simulink library "asbhl20vehicle"  (R2016b)
settings: Solver=ode45  StartTime=0.0  StopTime=10.0  RelTol=1e-3
undefined symbols (not defined in the file): alpha_vec_Cn0, b_ref, beta_vec_Cn0, Clbeta, Clda, Clddf, Cldr, Clp, Clr, Cm0, cm_GE, cm_LG, Cmda, Cmde, Cmdfn, Cmdfp, Cmdr, Cmq, Cn0, Cnda, Cnddf, Cndr, Cnp, Cnr, CX0, cx_GE, cx_LG, CXda, CXddf, CXde, CXdfn, CXdfp, CXdr, CYbeta, CYda, CYddf, CYdr, CZ0, cz_GE, cz_LG, CZda, CZde, CZdfn, CZdfp, CZdr, d_ref, Earth, Euler_0, heading0, LongLat0, mass, Tfg, Tplant, Ts, WGS84, x_cg, x_ref
libraries: aerolibtransform2 x6, aerolibconvert2 x4, aerolibasang x3, aerolibobsolete x3, aerolibutil x3, aerolib6dof2 x1, aerolibadyn x1, asbhl20act x1, discretizing x1
(part 1 of 2)
Description:
  | HL-20 vehicle plant model top component module (continuous)
settings Model: ExtModeAutoUpdateStatusClock=off  Creator=The MathWorks, Inc.  LastModifiedBy=The MathWorks, Inc.
settings DataIOCC: LimitDataPoints=on  SaveFormat=Array  SignalLoggingSaveFormat=ModelDataLogs
settings OptimizationCC: BlockReduction=off  BooleanDataType=off  ExpressionDepthLimit=2147483647  LifeSpan=inf
settings DebuggingCC: SaveWithParameterizedLinksMsg=none  UnderspecifiedInitializationDetection=Classic  MergeDetectMultiDrivingBlocksExec=none  SignalResolutionControl=TryResolveAllWithWarning  FcnCallInpInsideContextMsg=warning  StateNameClashWarn=warning  StrictBusMsg=Warning  SFUnexpectedBacktrackingDiag=warning  SFNoUnconditionalDefaultTransitionDiag=warning  SFExecutionAtInitializationDiag=none
settings HardwareCC: ProdBitPerPointer=32  ProdBitPerSizeT=32  ProdBitPerPtrDiffT=32  ProdLargestAtomicFloat=None  ProdIntDivRoundTo=Undefined  ProdEndianess=Unspecified  ProdWordSize=32  ProdHWDeviceType=32-bit Generic  TargetUnknown=on
settings ModelReferenceCC: PropagateSignalLabelsOutOfModel=off
settings GRTTargetCC: TargetLangStandard=C89/C90 (ANSI)  GeneratePreprocessorConditionals=Disable all  CombineOutputUpdateFcns=off  GRTInterface=on
settings ConfigComp: CovMetricSettings=dw  CovHtmlReporting=on  CovSaveCumulativeToWorkspaceVar=on  CovSaveSingleToWorkspaceVar=on  CovExternalEMLEnable=off

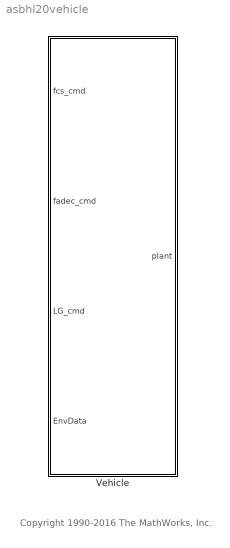
== system asbhl20vehicle ==
  note: Copyright 1990-2016 The MathWorks, Inc.
  Vehicle : Subsystem

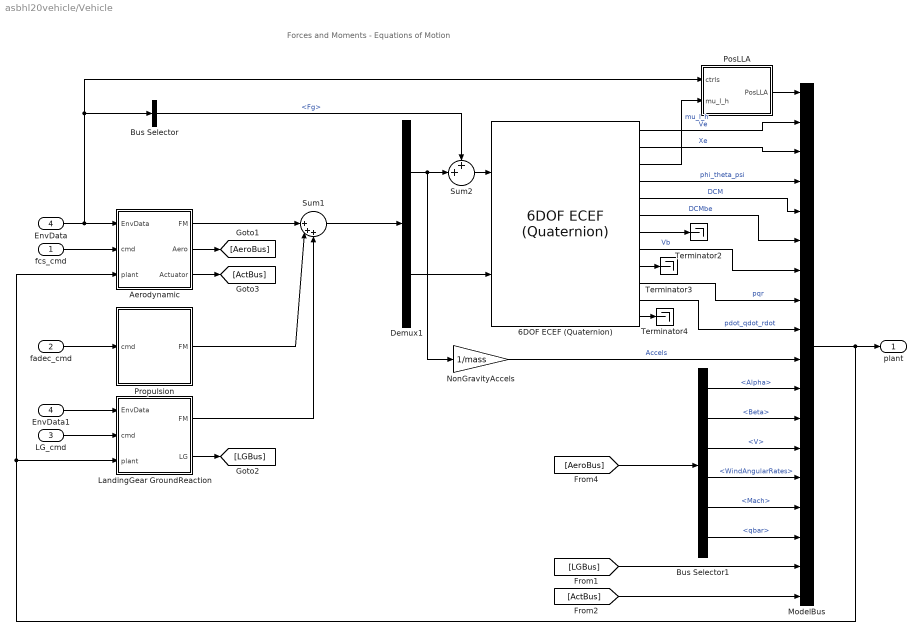
== system asbhl20vehicle/Vehicle ==
  note: Forces and Moments - Equations of Motion
  fcs_cmd : Inport
  fadec_cmd : Inport  Port=2
  LG_cmd : Inport  Port=3
  EnvData : Inport  Port=4
  6DOF ECEF (Quaternion) : aerolib6dof2/6DOF ECEF (Quaternion)  units=Metric (MKS)  mtype=Fixed  xg_0="[LongLat0(2)  LongLat0(1) 2275.5]"  Vm_0=Vmw  eul_0=[Euler_0(1) Euler_0(2) Euler_0(3)+heading0*pi/180]  pm_0=pm_0  mass_0=mass  mass_e=0.5  mass_f=2.0  inertia=Inertia  inertia_e=eye(3)  inertia_f=2*eye(3)  vre_flag=on  ptype=Earth (WGS84)  R=6378137  F=1/298.257223563  w_E=7292115e-11  angle_in=Internal  LG0=0
  Aerodynamic : Subsystem
  Bus Selector : BusSelector  OutputSignals=Fg
  Bus Selector1 : BusSelector  OutputSignals=Alpha,Beta,V,WindAngularRates,Mach,qbar
  Demux1 : Demux  Outputs=[3,3]
  EnvData1 : InportShadow  Port=4
  LandingGear GroundReaction : Subsystem
  ModelBus : BusCreator  Inputs='PosLLA','Ve','Xe','phi_theta_psi','DCM','DCMbe','Vb','pqr','pdot_qdot_rdot','Accels','Alpha','Beta','V','WindAngularRates','Mach','qbar','LGData','Act_positions'
  NonGravityAccels : Gain  Gain=1/mass  SaturateOnIntegerOverflow=on  OutDataTypeStr=Inherit: Same as input  ParamDataTypeStr=Inherit: Same as input
  PosLLA : Subsystem
  Propulsion : Subsystem  SystemSampleTime=Tfg
      settings: RTWSystemCode=Inline
  Sum1 : Sum  Inputs=||+++  SaturateOnIntegerOverflow=on  InputSameDT=on  OutDataTypeStr=Inherit: Same as first input
  Sum2 : Sum  Inputs=++|  SaturateOnIntegerOverflow=on  InputSameDT=on  OutDataTypeStr=Inherit: Same as first input
  Terminator2 : Terminator
  Terminator3 : Terminator
  Terminator4 : Terminator
  plant : Outport
  wires:
  PosLLA/1(PosLLA) -> ModelBus/1
  6DOF ECEF (Quaternion)/11 -> ModelBus/9  "pdot_qdot_rdot"
  6DOF ECEF (Quaternion)/12 -> Terminator4/1
  6DOF ECEF (Quaternion)/9 -> Terminator3/1
  6DOF ECEF (Quaternion)/10 -> ModelBus/8  "pqr"
  6DOF ECEF (Quaternion)/8 -> ModelBus/7  "Vb"
  6DOF ECEF (Quaternion)/7 -> Terminator2/1
  6DOF ECEF (Quaternion)/6 -> ModelBus/6  "DCMbe"
  6DOF ECEF (Quaternion)/5 -> ModelBus/5  "DCM"
  6DOF ECEF (Quaternion)/4 -> ModelBus/4  "phi_theta_psi"
  6DOF ECEF (Quaternion)/2 -> ModelBus/3  "Xe"
  6DOF ECEF (Quaternion)/1 -> ModelBus/2  "Ve"
  6DOF ECEF (Quaternion)/3 -> PosLLA/2(mu_l_h)  "mu_l_h"
  EnvData1/1 -> LandingGear GroundReaction/1(EnvData)
  Demux1/2 -> 6DOF ECEF (Quaternion)/2
  Aerodynamic/1(FM) -> Sum1/1
  LandingGear GroundReaction/1(FM) -> Sum1/3
  Sum1/1 -> Demux1/1
  EnvData/1 -> PosLLA/1(ctrls), Bus Selector/1, Aerodynamic/1(EnvData)
  fcs_cmd/1 -> Aerodynamic/2(cmd)
  fadec_cmd/1 -> Propulsion/1(cmd)
  Demux1/1 -> Sum2/2, NonGravityAccels/1
  Sum2/1 -> 6DOF ECEF (Quaternion)/1
  Bus Selector/1 -> Sum2/1  "<Fg>"
  NonGravityAccels/1 -> ModelBus/10  "Accels"
  Aerodynamic/2(Aero) -> [AeroBus]
  [AeroBus] -> Bus Selector1/1
  Bus Selector1/1 -> ModelBus/11  "<Alpha>"
  Bus Selector1/2 -> ModelBus/12  "<Beta>"
  Bus Selector1/3 -> ModelBus/13  "<V>"
  Bus Selector1/4 -> ModelBus/14  "<WindAngularRates>"
  Bus Selector1/5 -> ModelBus/15  "<Mach>"
  Bus Selector1/6 -> ModelBus/16  "<qbar>"
  LandingGear GroundReaction/2(LG) -> [LGBus]
  [LGBus] -> ModelBus/17
  LG_cmd/1 -> LandingGear GroundReaction/2(cmd)
  ModelBus/1 -> plant/1, Aerodynamic/3(plant), LandingGear GroundReaction/3(plant)
  Aerodynamic/3(Actuator) -> [ActBus]
  [ActBus] -> ModelBus/18
  Propulsion/1(FM) -> Sum1/2

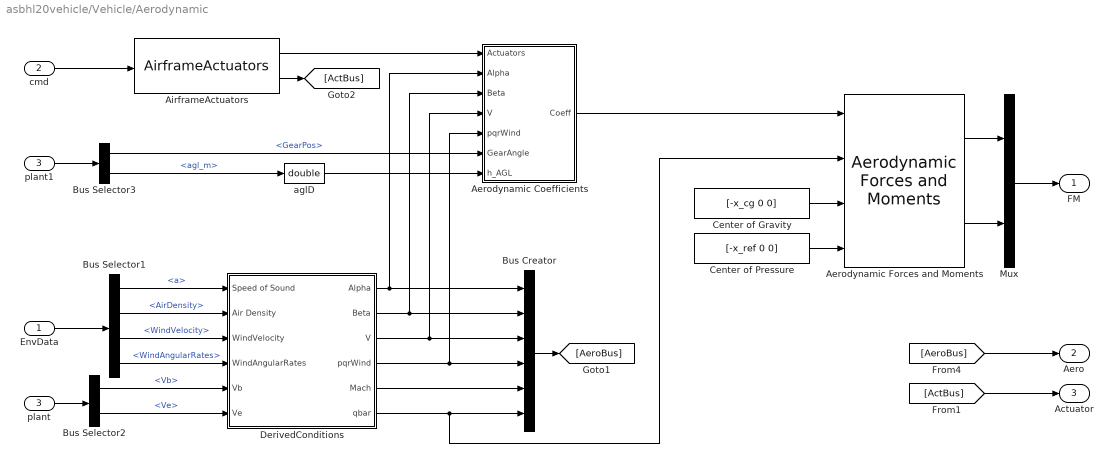
== system asbhl20vehicle/Vehicle/Aerodynamic ==
  EnvData : Inport
  cmd : Inport  Port=2
  plant : Inport  Port=3
  Aerodynamic Coefficients : Subsystem
  Aerodynamic Forces and Moments : aerolibadyn/Aerodynamic Forces and Moments   inputAxes=Body  outputForceAxes=Body  outputMomentAxes=Body  S=S_ref  b=b_ref  cbar=d_ref
  AirframeActuators : asbhl20act/AirframeActuators
  Bus Creator : BusCreator  Inputs='Alpha','Beta','V','WindAngularRates','Mach','qbar'
  Bus Selector1 : BusSelector  OutputSignals=a,AirDensity,WindVelocity,WindAngularRates
  Bus Selector2 : BusSelector  OutputSignals=Vb,Ve
  Bus Selector3 : BusSelector  OutputSignals=LGData.GearPos,PosLLA.agl_m
  Center of Gravity : Constant  Value=[-x_cg 0 0]  SampleTime=0
  Center of Pressure : Constant  Value=[-x_ref 0 0]  SampleTime=0
  DerivedConditions : Subsystem
  Mux : Mux  Inputs=2
  aglD : DataTypeConversion  OutDataTypeStr=double  SaturateOnIntegerOverflow=on
  plant1 : InportShadow  Port=3
  FM : Outport  PortDimensions=6  InitialOutput=0
  Aero : Outport  Port=2  InitialOutput=0
  Actuator : Outport  Port=3  InitialOutput=0
  wires:
  Center of Pressure/1 -> Aerodynamic Forces and Moments/4
  Center of Gravity/1 -> Aerodynamic Forces and Moments/3
  Bus Selector3/1 -> Aerodynamic Coefficients/6(GearAngle)  "<GearPos>"
  Bus Selector3/2 -> aglD/1  "<agl_m>"
  plant1/1 -> Bus Selector3/1
  cmd/1 -> AirframeActuators/1
  Aerodynamic Coefficients/1(Coeff) -> Aerodynamic Forces and Moments/1
  Aerodynamic Forces and Moments/1 -> Mux/1
  Aerodynamic Forces and Moments/2 -> Mux/2
  Mux/1 -> FM/1
  DerivedConditions/1(Alpha) -> Bus Creator/1, Aerodynamic Coefficients/2(Alpha)
  DerivedConditions/2(Beta) -> Bus Creator/2, Aerodynamic Coefficients/3(Beta)
  DerivedConditions/3(V) -> Bus Creator/3, Aerodynamic Coefficients/4(V)
  DerivedConditions/4("pqrWind ") -> Bus Creator/4, Aerodynamic Coefficients/5(pqrWind)
  DerivedConditions/5(Mach) -> Bus Creator/5
  DerivedConditions/6(qbar) -> Aerodynamic Forces and Moments/2, Bus Creator/6
  Bus Creator/1 -> [AeroBus]
  [AeroBus] -> Aero/1
  EnvData/1 -> Bus Selector1/1
  Bus Selector1/1 -> DerivedConditions/1(Speed of Sound)  "<a>"
  Bus Selector1/2 -> DerivedConditions/2(Air Density)  "<AirDensity>"
  plant/1 -> Bus Selector2/1
  Bus Selector1/3 -> DerivedConditions/3(WindVelocity)  "<WindVelocity>"
  Bus Selector1/4 -> DerivedConditions/4(WindAngularRates)  "<WindAngularRates>"
  AirframeActuators/1 -> Aerodynamic Coefficients/1(Actuators)
  Bus Selector2/1 -> DerivedConditions/5(Vb)  "<Vb>"
  Bus Selector2/2 -> DerivedConditions/6(Ve)  "<Ve>"
  aglD/1 -> Aerodynamic Coefficients/7(h_AGL)
  AirframeActuators/2 -> [ActBus]
  [ActBus] -> Actuator/1

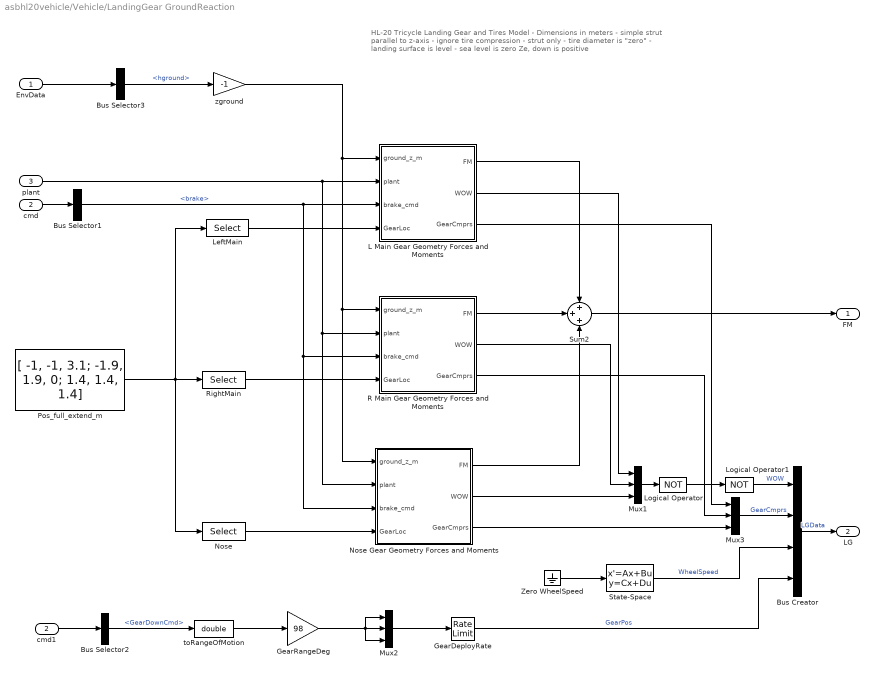
== system asbhl20vehicle/Vehicle/LandingGear GroundReaction ==
  note: HL-20 Tricycle Landing Gear and Tires Model
      |  - Dimensions in meters
      |  - simple strut parallel to z-axis
      |  - ignore tire compression - strut only
      |  - tire diameter is "zero"
      |  - landing surface is level
      |  - sea level is zero Ze, down is positive
  EnvData : Inport  SampleTime=Ts
  cmd : Inport  Port=2
  plant : Inport  Port=3
  Bus Creator : BusCreator  Inputs=4
  Bus Selector1 : BusSelector  OutputSignals=brake
  Bus Selector2 : BusSelector  OutputSignals=GearDownCmd
  Bus Selector3 : BusSelector  OutputSignals=hground
  GearDeployRate : RateLimiter  RisingSlewLimit=50  FallingSlewLimit=-50  SampleTimeMode=inherited
      settings: AttributesFormatString=[%<RisingSlewLimit>, %<FallingSlewLimit>] deg_per_sec
  GearRangeDeg : Gain  Gain=98
  L Main Gear Geometry Forces and Moments : Subsystem  TreatAsAtomicUnit=on
  LeftMain : Selector  NumberOfDimensions=2  InputPortWidth=3  IndexOptions=Select all,Index vector (dialog)  Indices=-1,1  OutputSizes=1
  Logical Operator : Logic  Operator=NOT  IconShape=distinctive  AllPortsSameDT=off  OutDataTypeStr=boolean
  Logical Operator1 : Logic  Operator=NOT  IconShape=distinctive  AllPortsSameDT=off  OutDataTypeStr=boolean
  Mux1 : Mux  Inputs=3
  Mux2 : Mux  Inputs=3
  Mux3 : Mux  Inputs=3
  Nose : Selector  NumberOfDimensions=2  InputPortWidth=3  IndexOptions=Select all,Index vector (dialog)  Indices=-1,3  OutputSizes=1
  Nose Gear Geometry Forces and Moments : Subsystem  TreatAsAtomicUnit=on
  Pos_full_extend_m : Constant  Description=|  Value=[ -1, -1, 3.1; -1.9, 1.9, 0; 1.4, 1.4, 1.4]
      | Rows are X, Y, Z; cols are Left, Right, Nose gear
      | Measured from CG in meters
      settings: AttributesFormatString=%<Description>
  R Main Gear Geometry Forces and Moments : Subsystem  TreatAsAtomicUnit=on
  RightMain : Selector  NumberOfDimensions=2  InputPortWidth=3  IndexOptions=Select all,Index vector (dialog)  Indices=-1,2  OutputSizes=1
  State-Space : StateSpace  A=[]  B=[]  C=[]  D=[1,1,1]'  X0=0
  Sum2 : Sum  Inputs=+++  SaturateOnIntegerOverflow=on  InputSameDT=on  OutDataTypeStr=Inherit: Same as first input
  Zero WheelSpeed : Ground
  cmd1 : InportShadow  Port=2
  toRangeOfMotion : DataTypeConversion  OutDataTypeStr=double  SampleTime=Tplant
  zground : Gain  Gain=-1
  FM : Outport
  LG : Outport  Port=2
  wires:
  Zero WheelSpeed/1 -> State-Space/1
  Logical Operator1/1 -> Bus Creator/1  "WOW"
  Logical Operator/1 -> Logical Operator1/1
  State-Space/1 -> Bus Creator/3  "WheelSpeed"
  Nose Gear Geometry Forces and Moments/3(GearCmprs) -> Mux3/3
  Mux3/1 -> Bus Creator/2  "GearCmprs"
  GearDeployRate/1 -> Bus Creator/4  "GearPos"
  R Main Gear Geometry Forces and Moments/3(GearCmprs) -> Mux3/2
  L Main Gear Geometry Forces and Moments/3(GearCmprs) -> Mux3/1
  Mux2/1 -> GearDeployRate/1
  GearRangeDeg/1 -> Mux2/3, Mux2/2, Mux2/1
  toRangeOfMotion/1 -> GearRangeDeg/1
  Bus Selector2/1 -> toRangeOfMotion/1  "<GearDownCmd>"
  cmd1/1 -> Bus Selector2/1
  Nose/1 -> Nose Gear Geometry Forces and Moments/4(GearLoc)
  Bus Selector1/1 -> Nose Gear Geometry Forces and Moments/3(brake_cmd), R Main Gear Geometry Forces and Moments/3(brake_cmd), L Main Gear Geometry Forces and Moments/3(brake_cmd)  "<brake>"
  RightMain/1 -> R Main Gear Geometry Forces and Moments/4(GearLoc)
  L Main Gear Geometry Forces and Moments/1(FM) -> Sum2/1
  Nose Gear Geometry Forces and Moments/2(WOW) -> Mux1/3
  R Main Gear Geometry Forces and Moments/2(WOW) -> Mux1/2
  L Main Gear Geometry Forces and Moments/2(WOW) -> Mux1/1
  Nose Gear Geometry Forces and Moments/1(FM) -> Sum2/3
  Sum2/1 -> FM/1
  R Main Gear Geometry Forces and Moments/1(FM) -> Sum2/2
  LeftMain/1 -> L Main Gear Geometry Forces and Moments/4(GearLoc)
  Pos_full_extend_m/1 -> LeftMain/1, Nose/1, RightMain/1
  zground/1 -> L Main Gear Geometry Forces and Moments/1(ground_z_m), Nose Gear Geometry Forces and Moments/1(ground_z_m), R Main Gear Geometry Forces and Moments/1(ground_z_m)
  Bus Selector3/1 -> zground/1  "<hground>"
  Mux1/1 -> Logical Operator/1
  cmd/1 -> Bus Selector1/1
  EnvData/1 -> Bus Selector3/1
  Bus Creator/1 -> LG/1  "LGData"
  plant/1 -> Nose Gear Geometry Forces and Moments/2(plant), R Main Gear Geometry Forces and Moments/2(plant), L Main Gear Geometry Forces and Moments/2(plant)

== system asbhl20vehicle/Vehicle/PosLLA ==
  ctrls : Inport
  mu_l_h : Inport  Port=2
  Bus Selector : BusSelector  OutputSignals=hground
  Demux1 : Demux  Outputs=2
  Demux2 : Demux  Outputs=[2 1]
  FilteredROC : discretizing/Discretized Transfer Fcn  Numerator=[1 0]  Denominator=[1 1]  AbsTol=auto  SampleTime=1.0  method=tustin  Wc=1
  ModelBus : BusCreator  Inputs='long_rad','lat_rad','agl_m','alt_m','roc_fps'
  Sel : Selector  InputPortWidth=2  IndexOptions=Index vector (dialog)  Indices=[2 1]  OutputSizes=1
  Sum1 : Sum  Inputs=-+|
  altm : DataTypeConversion  OutDataTypeStr=single  SaturateOnIntegerOverflow=on
  m2ft : aerolibconvert2/Length Conversion  IU=m  OU=ft
  pos_rad : aerolibconvert2/Angle Conversion  IU=deg  OU=rad
  rocF : DataTypeConversion  OutDataTypeStr=single  SaturateOnIntegerOverflow=on
  PosLLA : Outport
  wires:
  altm/1 -> Sum1/2
  Sum1/1 -> ModelBus/3  "agl_m"
  Bus Selector/1 -> Sum1/1  "<hground>"
  ctrls/1 -> Bus Selector/1
  Sel/1 -> pos_rad/1
  Demux2/1 -> Sel/1
  pos_rad/1 -> Demux1/1
  Demux1/1 -> ModelBus/1  "long_rad"
  Demux1/2 -> ModelBus/2  "lat_rad"
  Demux2/2 -> altm/1, m2ft/1, ModelBus/4  "alt_m"
  rocF/1 -> ModelBus/5  "roc_fps"
  mu_l_h/1 -> Demux2/1
  ModelBus/1 -> PosLLA/1  "PosLLA"
  m2ft/1 -> FilteredROC/1
  FilteredROC/1 -> rocF/1

== system asbhl20vehicle/Vehicle/Propulsion ==
  note: HL-20 Propulsion Model
      |   - Thrusters not modeled
  cmd : Inport  SampleTime=Ts
  Mux : Mux  Inputs=3
  SigCat : SignalConversion  ConversionOutput=Contiguous copy  OverrideOpt=off
  ThrustX : Lookup_n-D  NumberOfTableDimensions=1  BreakpointsForDimension1=(1/6)*(3+([-3:3]))  IndexSearchMethod=Linear search  BeginIndexSearchUsingPreviousIndexResult=on  Table=10000*(1+tanh([-3:3]))  ExtrapMethod=Clip  InputSameDT=on
  Thrust_LMN : Constant  Value=[0, 0, 0]  SampleTime=Ts
  Thrust_YZ : Constant  Value=[0, 0]  SampleTime=Ts
  FM : Outport  PortDimensions=6
  wires:
  ThrustX/1 -> Mux/1
  Thrust_YZ/1 -> Mux/2
  Mux/1 -> SigCat/1
  SigCat/1 -> FM/1
  cmd/1 -> ThrustX/1
  Thrust_LMN/1 -> Mux/3

== system asbhl20vehicle/Vehicle/Aerodynamic/Aerodynamic Coefficients ==
  Actuators : Inport
  Alpha : Inport  Port=2
  Beta : Inport  Port=3
  V : Inport  Port=4
  pqrWind : Inport  Port=5
  GearAngle : Inport  Port=6
  h_AGL : Inport  Port=7
  Actuator Increments : Subsystem
  Body Rate Damping : Subsystem
  Datum Coefficients : Subsystem
  Ground Effects : Subsystem
  Landing Gear Effects : Subsystem
  Sum1 : Sum  Inputs=+++  SaturateOnIntegerOverflow=on  InputSameDT=on  OutDataTypeStr=Inherit: Same as first input
  Sum2 : Sum  Inputs=+++  SaturateOnIntegerOverflow=on  InputSameDT=on  OutDataTypeStr=Inherit: Same as first input
  alpha_rad : aerolibconvert2/Angle Conversion  IU=rad  OU=deg
  beta_rad : aerolibconvert2/Angle Conversion  IU=rad  OU=deg
  on_off1 : Gain
  on_off2 : Gain
  Coeff : Outport  InitialOutput=0
  wires:
  on_off1/1 -> Sum2/3
  on_off2/1 -> Sum2/2
  Ground Effects/1(Coeff) -> on_off1/1
  Landing Gear Effects/1(Coeff) -> on_off2/1
  Sum1/1 -> Sum2/1
  Sum2/1 -> Coeff/1
  GearAngle/1 -> Landing Gear Effects/3(Landing Gear Angle)
  h_AGL/1 -> Ground Effects/3(h_AGL)
  Body Rate Damping/1(cl) -> Sum1/3
  Actuator Increments/1(cl) -> Sum1/1
  V/1 -> Body Rate Damping/1(V)
  Beta/1 -> beta_rad/1
  beta_rad/1 -> Ground Effects/2(Beta), Landing Gear Effects/2(Beta), Datum Coefficients/2(Beta), Actuator Increments/2(Beta)
  Datum Coefficients/1(cl) -> Sum1/2
  Actuators/1 -> Actuator Increments/3("Actuator Deflections ")
  Alpha/1 -> alpha_rad/1
  pqrWind/1 -> Body Rate Damping/2(p,q,r)
  alpha_rad/1 -> Ground Effects/1(Alpha), Landing Gear Effects/1(Alpha), Body Rate Damping/3(Alpha), Datum Coefficients/1(Alpha), Actuator Increments/1(Alpha)

== system asbhl20vehicle/Vehicle/Aerodynamic/DerivedConditions ==
  note: TODO: clean up interface
  Speed of Sound : Inport
  Air Density : Inport  Port=2
  WindVelocity : Inport  Port=3  PortDimensions=3
  WindAngularRates : Inport  Port=4  PortDimensions=3
  Vb : Inport  Port=5  PortDimensions=3
  Ve : Inport  Port=6  PortDimensions=3
  Dynamic Pressure : aerolibasang/Dynamic Pressure
  "Incidence, Sideslip, & Airspeed" : aerolibasang/Incidence, Sideslip, & Airspeed
  Mach Number : aerolibasang/Mach Number
  Sum2 : Sum  Inputs=|+-  SaturateOnIntegerOverflow=on  InputSameDT=on  OutDataTypeStr=Inherit: Same as first input
  Terminator : Terminator
  Alpha : Outport
  Beta : Outport  Port=2
  V : Outport  Port=3
  "pqrWind " : Outport  Port=4
  Mach : Outport  Port=5
  qbar : Outport  Port=6  InitialOutput=0
  wires:
  "Incidence, Sideslip, & Airspeed"/1 -> Alpha/1  "Alpha"
  "Incidence, Sideslip, & Airspeed"/2 -> Beta/1  "Beta"
  Speed of Sound/1 -> Mach Number/2
  "Incidence, Sideslip, & Airspeed"/3 -> V/1  "V"
  Mach Number/1 -> Mach/1  "Mach"
  Air Density/1 -> Dynamic Pressure/2
  Dynamic Pressure/1 -> qbar/1  "qbar"
  WindAngularRates/1 -> "pqrWind "/1
  Vb/1 -> Sum2/1
  Sum2/1 -> Dynamic Pressure/1, Mach Number/1, "Incidence, Sideslip, & Airspeed"/1
  WindVelocity/1 -> Sum2/2
  Ve/1 -> Terminator/1

== system asbhl20vehicle/Vehicle/LandingGear GroundReaction/L Main Gear Geometry Forces and Moments ==
  note: Gear compression is assumed to occur
      | algebraically in proportion to the amount
      | of fully extended gear that would be
      | "below ground".
  note: HL-20 Tricycle Landing Gear and Tires Model
      |  - Dimensions in meters
      |  - simple strut parallel to z-axis
      |  - ignore tire compression - strut only
      |  - landing surface is level
      |  - sea level is zero Ze, down is positive
  ground_z_m : Inport
  plant : Inport  Port=2
  brake_cmd : Inport  Port=3
  GearLoc : Inport  Port=4
  Bus Selector3 : BusSelector  OutputSignals=PosLLA.alt_m,phi_theta_psi
  GearLoc1 : InportShadow  Port=4
  GenerateGroundFM : Subsystem  TreatAsAtomicUnit=on
  Rotate pos to body axes : Product  Multiplication=Matrix(*)  SaturateOnIntegerOverflow=on  InputSameDT=on  OutDataTypeStr=Inherit: Same as first input
  Subsystem : Subsystem
  Sum3 : Sum  Inputs=-+
  Zg : Selector  InputPortWidth=3  IndexOptions=Index vector (dialog)  Indices=3  OutputSizes=1
  detect_WOW : RelationalOperator  OutDataTypeStr=boolean  RndMeth=Nearest
  FM : Outport  PortDimensions=6
  WOW : Outport  Port=2
  GearCmprs : Outport  Port=3
  wires:
  Bus Selector3/2 -> Subsystem/1(Euler)  "<phi_theta_psi>"
  Zg/1 -> Sum3/2
  GenerateGroundFM/2(GearCmprs) -> GearCmprs/1
  Bus Selector3/1 -> [Xe]  "<alt_m>"
  [ZcL] -> GenerateGroundFM/2(ZcL)
  GenerateGroundFM/1(FM) -> FM/1
  brake_cmd/1 -> GenerateGroundFM/4(BrakeCmd)
  GearLoc1/1 -> Rotate pos to body axes/2
  [DCM] -> Rotate pos to body axes/1
  plant/1 -> Bus Selector3/1, GenerateGroundFM/3(plant)
  GearLoc/1 -> GenerateGroundFM/5(GearLoc)
  ground_z_m/1 -> detect_WOW/2, GenerateGroundFM/1(ground_z)
  detect_WOW/1 -> WOW/1, GenerateGroundFM/Enable
  Rotate pos to body axes/1 -> Zg/1
  Sum3/1 -> detect_WOW/1
  [Xe] -> [ZcL], Sum3/1
  Subsystem/1(DCM) -> [DCM]

== system asbhl20vehicle/Vehicle/LandingGear GroundReaction/Nose Gear Geometry Forces and Moments ==
  note: Gear compression is assumed to occur
      | algebraically in proportion to the amount
      | of fully extended gear that would be
      | "below ground".
  note: HL-20 Tricycle Landing Gear and Tires Model
      |  - Dimensions in meters
      |  - simple strut parallel to z-axis
      |  - ignore tire compression - strut only
      |  - landing surface is level
      |  - sea level is zero Ze, down is positive
  ground_z_m : Inport
  plant : Inport  Port=2
  brake_cmd : Inport  Port=3
  GearLoc : Inport  Port=4
  Bus Selector3 : BusSelector  OutputSignals=PosLLA.alt_m,phi_theta_psi
  GearLoc1 : InportShadow  Port=4
  GenerateGroundFM : Subsystem  TreatAsAtomicUnit=on
  Rotate pos to body axes : Product  Multiplication=Matrix(*)  SaturateOnIntegerOverflow=on  InputSameDT=on  OutDataTypeStr=Inherit: Same as first input
  Subsystem : Subsystem
  Sum3 : Sum  Inputs=-+
  Zg : Selector  InputPortWidth=3  IndexOptions=Index vector (dialog)  Indices=3  OutputSizes=1
  detect_WOW : RelationalOperator  OutDataTypeStr=boolean  RndMeth=Nearest
  FM : Outport  PortDimensions=6
  WOW : Outport  Port=2
  GearCmprs : Outport  Port=3
  wires:
  Zg/1 -> Sum3/2
  GenerateGroundFM/2(GearCmprs) -> GearCmprs/1
  Bus Selector3/1 -> [Xe]  "<alt_m>"
  [ZcL] -> GenerateGroundFM/2(ZcL)
  GenerateGroundFM/1(FM) -> FM/1
  brake_cmd/1 -> GenerateGroundFM/4(BrakeCmd)
  GearLoc1/1 -> Rotate pos to body axes/2
  [DCM] -> Rotate pos to body axes/1
  plant/1 -> Bus Selector3/1, GenerateGroundFM/3(plant)
  GearLoc/1 -> GenerateGroundFM/5(GearLoc)
  ground_z_m/1 -> GenerateGroundFM/1(ground_z), detect_WOW/2
  detect_WOW/1 -> GenerateGroundFM/Enable, WOW/1
  Rotate pos to body axes/1 -> Zg/1
  Sum3/1 -> detect_WOW/1
  [Xe] -> [ZcL], Sum3/1
  Bus Selector3/2 -> Subsystem/1(Euler)  "<phi_theta_psi>"
  Subsystem/1(DCM) -> [DCM]

== system asbhl20vehicle/Vehicle/LandingGear GroundReaction/R Main Gear Geometry Forces and Moments ==
  note: HL-20 Tricycle Landing Gear and Tires Model
      |  - Dimensions in meters
      |  - simple strut parallel to z-axis
      |  - ignore tire compression - strut only
      |  - landing surface is level
      |  - sea level is zero Ze, down is positive
  note: Gear compression is assumed to occur
      | algebraically in proportion to the amount
      | of fully extended gear that would be
      | "below ground".
  ground_z_m : Inport
  plant : Inport  Port=2
  brake_cmd : Inport  Port=3
  GearLoc : Inport  Port=4
  Bus Selector3 : BusSelector  OutputSignals=PosLLA.alt_m,phi_theta_psi
  GearLoc1 : InportShadow  Port=4
  GenerateGroundFM : Subsystem  TreatAsAtomicUnit=on
  Rotate pos to body axes : Product  Multiplication=Matrix(*)  SaturateOnIntegerOverflow=on  InputSameDT=on  OutDataTypeStr=Inherit: Same as first input
  Subsystem1 : Subsystem
  Sum3 : Sum  Inputs=-+
  Zg : Selector  InputPortWidth=3  IndexOptions=Index vector (dialog)  Indices=3  OutputSizes=1
  detect_WOW : RelationalOperator  OutDataTypeStr=boolean  RndMeth=Nearest
  FM : Outport  PortDimensions=6
  WOW : Outport  Port=2
  GearCmprs : Outport  Port=3
  wires:
  Subsystem1/1(DCM) -> [DCM]
  Zg/1 -> Sum3/2
  [Xe] -> [ZcL], Sum3/1
  Sum3/1 -> detect_WOW/1
  Rotate pos to body axes/1 -> Zg/1
  detect_WOW/1 -> GenerateGroundFM/Enable, WOW/1
  ground_z_m/1 -> detect_WOW/2, GenerateGroundFM/1(ground_z)
  GearLoc/1 -> GenerateGroundFM/5(GearLoc)
  plant/1 -> GenerateGroundFM/3(plant), Bus Selector3/1
  [DCM] -> Rotate pos to body axes/1
  GearLoc1/1 -> Rotate pos to body axes/2
  brake_cmd/1 -> GenerateGroundFM/4(BrakeCmd)
  GenerateGroundFM/1(FM) -> FM/1
  [ZcL] -> GenerateGroundFM/2(ZcL)
  Bus Selector3/1 -> [Xe]  "<alt_m>"
  GenerateGroundFM/2(GearCmprs) -> GearCmprs/1
  Bus Selector3/2 -> Subsystem1/1(Euler)  "<phi_theta_psi>"

== system asbhl20vehicle/Vehicle/Aerodynamic/Aerodynamic Coefficients/Actuator Increments ==
  Alpha : Inport
  Beta : Inport  Port=2
  "Actuator Deflections " : Inport  Port=3
  (0 to inf) Constants Held fixed for alpha<0 : Saturate  UpperLimit=inf  LowerLimit=0
  Aileron : Subsystem
  AlphaLookup : PreLookup  BreakpointsData=alpha_vec_0  BeginIndexSearchUsingPreviousIndexResult=on  ExtrapMethod=Linear
  AlphaLookup0 : PreLookup  BreakpointsData=alpha_vec_0  BeginIndexSearchUsingPreviousIndexResult=on  ExtrapMethod=Linear
  Bus Creator : BusCreator  Inputs=2
  Bus Creator1 : BusCreator  Inputs=2
  Elevator : Subsystem
  Flap(diff) : Subsystem
  Flap(neg) : Subsystem
  Flap(pos) : Subsystem
  Rudder : Subsystem
  Sum : Sum  Inputs=++++++  SaturateOnIntegerOverflow=on  InputSameDT=on  OutDataTypeStr=Inherit: Same as first input
  Terminator1 : Terminator
  cl : Outport  InitialOutput=0
  wires:
  Bus Creator/1 -> Aileron/1(Alpha), Rudder/1(Alpha)
  (0 to inf) Constants Held fixed for alpha<0/1 -> AlphaLookup0/1
  "Actuator Deflections "/1 -> Aileron/2(Actuators), Elevator/2(Actuators), Rudder/2(Actuators), Flap(pos)/2(Actuators), Flap(neg)/2(Actuators), Flap(diff)/2(Actuators)
  Alpha/1 -> (0 to inf) Constants Held fixed for alpha<0/1, AlphaLookup/1
  Beta/1 -> Terminator1/1
  Aileron/1(delCoeff) -> Sum/1
  Elevator/1(delCoeff) -> Sum/2
  Rudder/1(delCoeff) -> Sum/3
  Flap(pos)/1(delCoeff) -> Sum/4
  Flap(neg)/1(delCoeff) -> Sum/5
  Flap(diff)/1(delCoeff) -> Sum/6
  Sum/1 -> cl/1
  Bus Creator1/1 -> Flap(diff)/1(Alpha), Flap(neg)/1(Alpha), Flap(pos)/1(Alpha), Elevator/1(Alpha)
  AlphaLookup0/1 -> Bus Creator/1  "k"
  AlphaLookup0/2 -> Bus Creator/2  "f"
  AlphaLookup/1 -> Bus Creator1/1  "k"
  AlphaLookup/2 -> Bus Creator1/2  "f"

== system asbhl20vehicle/Vehicle/Aerodynamic/Aerodynamic Coefficients/Body Rate Damping ==
  V : Inport
  p,q,r : Inport  Port=2
  Alpha : Inport  Port=3
  AlphaLookup : PreLookup  BreakpointsData=alpha_vec_damping  BeginIndexSearchUsingPreviousIndexResult=on  ExtrapMethod=Linear
  Bus Creator : BusCreator  Inputs=2
  Demux : Demux  Outputs=3
  Product : Product  SaturateOnIntegerOverflow=on  InputSameDT=on  OutDataTypeStr=Inherit: Same as first input
  Product1 : Product  SaturateOnIntegerOverflow=on  InputSameDT=on  OutDataTypeStr=Inherit: Same as first input
  Product2 : Product  SaturateOnIntegerOverflow=on  InputSameDT=on  OutDataTypeStr=Inherit: Same as first input
  Product3 : Product  Inputs=*/  SaturateOnIntegerOverflow=on  InputSameDT=on  OutDataTypeStr=Inherit: Same as first input
  Reference Length : Gain  Gain=d_ref/2  SaturateOnIntegerOverflow=on  OutDataTypeStr=Inherit: Same as input  ParamDataTypeStr=Inherit: Same as input
  Reference Span : Gain  Gain=b_ref/2  SaturateOnIntegerOverflow=on  OutDataTypeStr=Inherit: Same as input  ParamDataTypeStr=Inherit: Same as input
  "Reference Span " : Gain  Gain=b_ref/2  SaturateOnIntegerOverflow=on  OutDataTypeStr=Inherit: Same as input  ParamDataTypeStr=Inherit: Same as input
  Sum1 : Sum  Inputs=+++  SaturateOnIntegerOverflow=on  InputSameDT=on  OutDataTypeStr=Inherit: Same as first input
  p : Subsystem
  q : Subsystem
  r : Subsystem
  cl : Outport  InitialOutput=0
  wires:
  Alpha/1 -> AlphaLookup/1
  p/1(delCoeff) -> Product/1
  q/1(delCoeff) -> Product1/1
  p,q,r/1 -> Demux/1
  Demux/1 -> Product/2  "p"
  Demux/2 -> Product1/2  "q"
  Demux/3 -> Product2/2  "r"
  Sum1/1 -> Product3/1
  V/1 -> Product3/2
  Product3/1 -> cl/1
  Product1/1 -> Reference Length/1
  Product2/1 -> "Reference Span "/1
  Product/1 -> Reference Span/1
  r/1(delCoeff) -> Product2/1
  Bus Creator/1 -> r/1(Alpha), q/1(Alpha), p/1(Alpha)
  Reference Length/1 -> Sum1/2
  Reference Span/1 -> Sum1/1
  "Reference Span "/1 -> Sum1/3
  AlphaLookup/1 -> Bus Creator/1  "k"
  AlphaLookup/2 -> Bus Creator/2  "f"

== system asbhl20vehicle/Vehicle/Aerodynamic/Aerodynamic Coefficients/Datum Coefficients ==
  Alpha : Inport
  Beta : Inport  Port=2
  " Cn" : Lookup_n-D  BreakpointsForDimension1=alpha_vec_Cn0  BreakpointsForDimension2=beta_vec_Cn0  Table=Cn0  InternalRulePriority=Speed  RndMeth=Simplest  InputSameDT=on
  " Beta" : InportShadow  Port=2
  " Beta " : InportShadow  Port=2
  Abs : Abs  SaturateOnIntegerOverflow=on
  "Alpha " : InportShadow
  AlphaLookup : PreLookup  BreakpointsData=alpha_vec_0  BeginIndexSearchUsingPreviousIndexResult=on  ExtrapMethod=Linear
  "Beta " : InportShadow  Port=2
  BetaLookup : PreLookup  BreakpointsData=beta_vec_0  BeginIndexSearchUsingPreviousIndexResult=on  ExtrapMethod=Linear
  Cl : Gain  Gain=Clbeta  SaturateOnIntegerOverflow=on  OutDataTypeStr=Inherit: Same as input  ParamDataTypeStr=Inherit: Same as input
  Cm : Interpolation_n-D  Table=Cm0'  RemoveProtectionIndex=on  SaturateOnIntegerOverflow=on
  Cx : Interpolation_n-D  Table=CX0'  RemoveProtectionIndex=on  SaturateOnIntegerOverflow=on
  Cy : Gain  Gain=CYbeta  SaturateOnIntegerOverflow=on  OutDataTypeStr=Inherit: Same as input  ParamDataTypeStr=Inherit: Same as input
  Cz : Interpolation_n-D  Table=CZ0'  RemoveProtectionIndex=on  SaturateOnIntegerOverflow=on
  Mux1 : Mux  Inputs=6
  Product : Product  SaturateOnIntegerOverflow=on  InputSameDT=on  OutDataTypeStr=Inherit: Same as first input
  Sign : Signum
  cl : Outport  InitialOutput=0
  wires:
  Sign/1 -> Product/2
  " Cn"/1 -> Product/1
  Product/1 -> Mux1/6
  Abs/1 -> " Cn"/2
  Mux1/1 -> cl/1
  Cx/1 -> Mux1/1
  Cz/1 -> Mux1/3
  Cm/1 -> Mux1/5
  Cy/1 -> Mux1/2
  Cl/1 -> Mux1/4
  Alpha/1 -> AlphaLookup/1
  Beta/1 -> BetaLookup/1
  AlphaLookup/1 -> Cz/1, Cm/1, Cx/1
  BetaLookup/1 -> Cz/3, Cx/3, Cm/3
  AlphaLookup/2 -> Cx/2, Cm/2, Cz/2
  "Beta "/1 -> Cy/1
  "Alpha "/1 -> " Cn"/1
  " Beta"/1 -> Abs/1, Sign/1
  " Beta "/1 -> Cl/1
  BetaLookup/2 -> Cz/4, Cx/4, Cm/4

== system asbhl20vehicle/Vehicle/Aerodynamic/Aerodynamic Coefficients/Ground Effects ==
  Alpha : Inport
  Beta : Inport  Port=2
  h_AGL : Inport  Port=3
  AlphaLookup : PreLookup  BreakpointsData=GE_alpha_bp  BeginIndexSearchUsingPreviousIndexResult=on
  AltitudeLookup : PreLookup  BreakpointsData=GE_alt_bp  BeginIndexSearchUsingPreviousIndexResult=on
  Cm : Interpolation_n-D  Table=cm_GE  RemoveProtectionIndex=on  SaturateOnIntegerOverflow=on
  Constant1 : Constant  Value=0
  Constant2 : Constant  Value=0
  Constant3 : Constant  Value=0
  Cx : Interpolation_n-D  Table=cx_GE  RemoveProtectionIndex=on  SaturateOnIntegerOverflow=on
  Cz : Interpolation_n-D  Table=cz_GE  RemoveProtectionIndex=on  SaturateOnIntegerOverflow=on
  Gain : Gain  Gain=1/b_ref  SaturateOnIntegerOverflow=on  OutDataTypeStr=Inherit: Same as input  ParamDataTypeStr=Inherit: Same as input
  Mux1 : Mux  Inputs=6
  Terminator1 : Terminator
  Coeff : Outport
  wires:
  AltitudeLookup/2 -> Cm/4, Cz/4, Cx/4
  AlphaLookup/2 -> Cm/2, Cz/2, Cx/2
  Constant3/1 -> Mux1/6
  Cm/1 -> Mux1/5
  Constant2/1 -> Mux1/4
  Cz/1 -> Mux1/3
  Constant1/1 -> Mux1/2
  Cx/1 -> Mux1/1
  Mux1/1 -> Coeff/1
  h_AGL/1 -> Gain/1
  AlphaLookup/1 -> Cx/1, Cm/1, Cz/1
  Beta/1 -> Terminator1/1
  Alpha/1 -> AlphaLookup/1
  AltitudeLookup/1 -> Cm/3, Cz/3, Cx/3
  Gain/1 -> AltitudeLookup/1

== system asbhl20vehicle/Vehicle/Aerodynamic/Aerodynamic Coefficients/Landing Gear Effects ==
  Alpha : Inport
  Beta : Inport  Port=2
  Landing Gear Angle : Inport  Port=3
  AlphaLookup : PreLookup  BreakpointsData=LG_alpha_bp  BeginIndexSearchUsingPreviousIndexResult=on  ExtrapMethod=Linear
  Cm : Interpolation_n-D  Table=cm_LG  RemoveProtectionIndex=on  SaturateOnIntegerOverflow=on
  Constant1 : Constant  Value=0
  Constant2 : Constant  Value=0
  Constant3 : Constant  Value=0
  Cx : Interpolation_n-D  Table=cx_LG  RemoveProtectionIndex=on  SaturateOnIntegerOverflow=on
  Cz : Interpolation_n-D  Table=cz_LG  RemoveProtectionIndex=on  SaturateOnIntegerOverflow=on
  LGLookup : PreLookup  BreakpointsData=LG_bp  BeginIndexSearchUsingPreviousIndexResult=on  ExtrapMethod=Linear
  Mux1 : Mux  Inputs=6
  Sum of Elements : Sum  Inputs=+
  Terminator1 : Terminator
  avg : Gain  Gain=1/3
  Coeff : Outport
  wires:
  LGLookup/2 -> Cm/4, Cz/4, Cx/4
  AlphaLookup/2 -> Cm/2, Cx/2, Cz/2
  LGLookup/1 -> Cm/3, Cz/3, Cx/3
  Constant3/1 -> Mux1/6
  Cm/1 -> Mux1/5
  Constant2/1 -> Mux1/4
  Cz/1 -> Mux1/3
  Constant1/1 -> Mux1/2
  Cx/1 -> Mux1/1
  Mux1/1 -> Coeff/1
  Landing Gear Angle/1 -> Sum of Elements/1
  AlphaLookup/1 -> Cx/1, Cm/1, Cz/1
  Beta/1 -> Terminator1/1
  Alpha/1 -> AlphaLookup/1
  Sum of Elements/1 -> avg/1
  avg/1 -> LGLookup/1

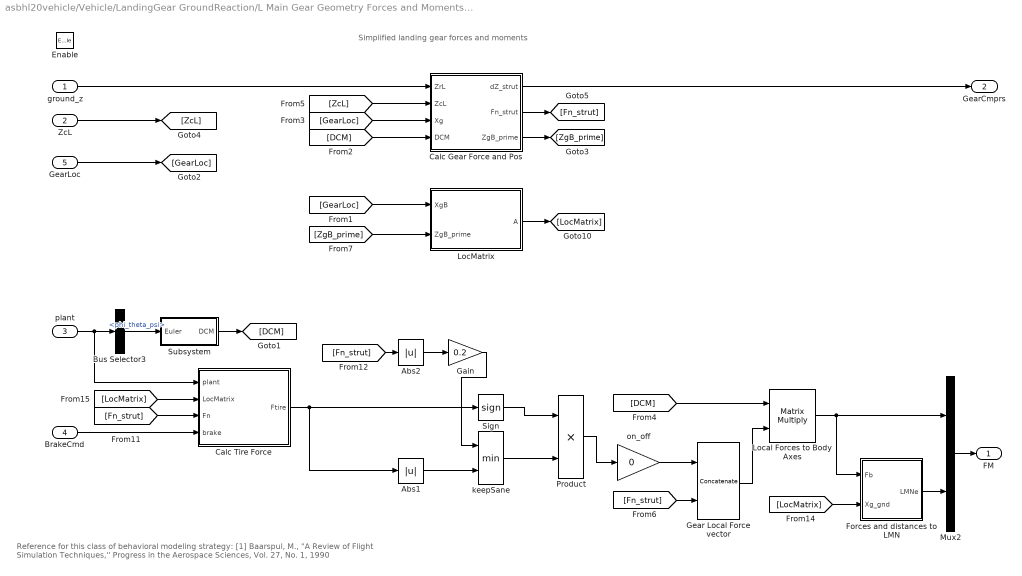
== system asbhl20vehicle/Vehicle/LandingGear GroundReaction/L Main Gear Geometry Forces and Moments/GenerateGroundFM ==
  note: Simplified landing gear forces and moments
  note: Reference for this class of behavioral modeling strategy:
      |
      | [1] Baarspul, M., "A Review of Flight Simulation Techniques,''
      | Progress in the Aerospace Sciences, Vol. 27, No. 1, 1990
  ground_z : Inport
  ZcL : Inport  Port=2
  plant : Inport  Port=3
  BrakeCmd : Inport  Port=4
  GearLoc : Inport  Port=5
  Enable : EnablePort  StatesWhenEnabling=reset
  Abs1 : Abs
  Abs2 : Abs
  Bus Selector3 : BusSelector  OutputSignals=phi_theta_psi
  Calc Gear Force and Pos : Subsystem
  Calc Tire Force : Subsystem
  Forces and distances to LMN : Subsystem
  Gain : Gain  Gain=0.2
  Gear Local Force vector : Concatenate  Mode=Multidimensional array
  LocMatrix : Subsystem
  Local Forces to Body Axes : Product  Multiplication=Matrix(*)  SaturateOnIntegerOverflow=on  InputSameDT=on  OutDataTypeStr=Inherit: Same as first input
  Mux2 : Mux  Inputs=2
  Product : Product  RndMeth=Zero
  Sign : Signum
  Subsystem : Subsystem
  keepSane : MinMax  Inputs=2
  on_off : Gain  Gain=0
  FM : Outport  PortDimensions=6  OutputWhenDisabled=reset  InitialOutput=[0,0,0,0,0,0]
  GearCmprs : Outport  Port=2  OutputWhenDisabled=reset  InitialOutput=0
  wires:
  ZcL/1 -> [ZcL]
  GearLoc/1 -> [GearLoc]
  Mux2/1 -> FM/1
  BrakeCmd/1 -> Calc Tire Force/4(brake)
  plant/1 -> Bus Selector3/1, Calc Tire Force/1(plant)
  ground_z/1 -> Calc Gear Force and Pos/1(ZrL)
  Calc Gear Force and Pos/1(dZ_strut) -> GearCmprs/1
  Sign/1 -> Product/1
  Product/1 -> on_off/1
  keepSane/1 -> Product/2
  Abs1/1 -> keepSane/2
  Gain/1 -> keepSane/1
  Abs2/1 -> Gain/1
  [Fn_strut] -> Abs2/1
  on_off/1 -> Gear Local Force vector/1
  Calc Tire Force/1(Ftire) -> Sign/1, Abs1/1
  [Fn_strut] -> Calc Tire Force/3(Fn)
  [LocMatrix] -> Calc Tire Force/2(LocMatrix)
  [LocMatrix] -> Forces and distances to LMN/2(Xg_gnd)
  LocMatrix/1(A) -> [LocMatrix]
  [ZgB_prime] -> LocMatrix/2(ZgB_prime)
  [GearLoc] -> LocMatrix/1(XgB)
  Forces and distances to LMN/1(LMNe) -> Mux2/2
  Gear Local Force vector/1 -> Local Forces to Body Axes/2
  [Fn_strut] -> Gear Local Force vector/2
  Local Forces to Body Axes/1 -> Mux2/1, Forces and distances to LMN/1(Fb)
  [DCM] -> Local Forces to Body Axes/1
  [DCM] -> Calc Gear Force and Pos/4(DCM)
  [GearLoc] -> Calc Gear Force and Pos/3(Xg)
  Calc Gear Force and Pos/2(Fn_strut) -> [Fn_strut]
  [ZcL] -> Calc Gear Force and Pos/2(ZcL)
  Calc Gear Force and Pos/3(ZgB_prime) -> [ZgB_prime]
  Bus Selector3/1 -> Subsystem/1(Euler)  "<phi_theta_psi>"
  Subsystem/1(DCM) -> [DCM]

== system asbhl20vehicle/Vehicle/LandingGear GroundReaction/L Main Gear Geometry Forces and Moments/Subsystem ==
  Euler : Inport
  Bias : Bias  Bias=[0.0 0.0 -heading0*pi/180]
  Rotation Angles to Direction Cosine Matrix : aerolibtransform2/Rotation Angles to Direction Cosine Matrix  rotationOrder=ZYX
  Selector : Selector  InputPortWidth=3  IndexOptions=Index vector (dialog)  Indices=[3 2 1]  OutputSizes=1
  DCM : Outport
  wires:
  Bias/1 -> Selector/1
  Euler/1 -> Bias/1
  Rotation Angles to Direction Cosine Matrix/1 -> DCM/1
  Selector/1 -> Rotation Angles to Direction Cosine Matrix/1

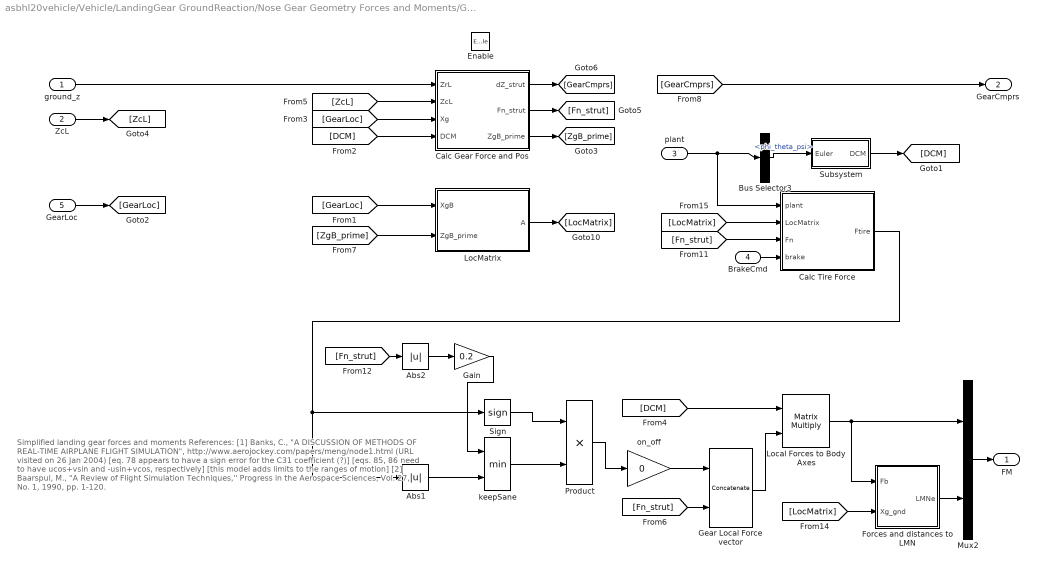
== system asbhl20vehicle/Vehicle/LandingGear GroundReaction/Nose Gear Geometry Forces and Moments/GenerateGroundFM ==
  note: Simplified landing gear forces and moments
      |
      | References:
      |
      | [1] Banks, C., "A DISCUSSION OF METHODS OF REAL-TIME AIRPLANE FLIGHT SIMULATION",
      | http://www.aerojockey.com/papers/meng/node1.html (URL visited on 26 Jan 2004)
      | [eq. 78 appears to have a sign error for the C31 coefficient (?)]
      | [eqs. 85, 86 need to have ucos+vsin and -usin+vcos, respectively]
      | [this model adds limits to the ranges of motion]
      |
      | [2] Baarspul, M., "A Review of Flight Simulation Techniques,''
      | Progress in the Aerospace Sciences, Vol. 27, No. 1, 1990, pp. 1-120.
  ground_z : Inport
  ZcL : Inport  Port=2
  plant : Inport  Port=3
  BrakeCmd : Inport  Port=4
  GearLoc : Inport  Port=5
  Enable : EnablePort  StatesWhenEnabling=reset
  Abs1 : Abs
  Abs2 : Abs
  Bus Selector3 : BusSelector  OutputSignals=phi_theta_psi
  Calc Gear Force and Pos : Subsystem
  Calc Tire Force : Subsystem
  Forces and distances to LMN : Subsystem
  Gain : Gain  Gain=0.2
  Gear Local Force vector : Concatenate  Mode=Multidimensional array
  LocMatrix : Subsystem
  Local Forces to Body Axes : Product  Multiplication=Matrix(*)  SaturateOnIntegerOverflow=on  InputSameDT=on  OutDataTypeStr=Inherit: Same as first input
  Mux2 : Mux  Inputs=2
  Product : Product  RndMeth=Zero
  Sign : Signum
  Subsystem : Subsystem
  keepSane : MinMax  Inputs=2
  on_off : Gain  Gain=0
  FM : Outport  PortDimensions=6  OutputWhenDisabled=reset  InitialOutput=[0,0,0,0,0,0]
  GearCmprs : Outport  Port=2  OutputWhenDisabled=reset  InitialOutput=0
  wires:
  [GearCmprs] -> GearCmprs/1
  ZcL/1 -> [ZcL]
  GearLoc/1 -> [GearLoc]
  Mux2/1 -> FM/1
  BrakeCmd/1 -> Calc Tire Force/4(brake)
  plant/1 -> Bus Selector3/1, Calc Tire Force/1(plant)
  ground_z/1 -> Calc Gear Force and Pos/1(ZrL)
  Calc Gear Force and Pos/1(dZ_strut) -> [GearCmprs]
  Sign/1 -> Product/1
  Product/1 -> on_off/1
  keepSane/1 -> Product/2
  Abs1/1 -> keepSane/2
  Gain/1 -> keepSane/1
  Abs2/1 -> Gain/1
  [Fn_strut] -> Abs2/1
  on_off/1 -> Gear Local Force vector/1
  Calc Tire Force/1(Ftire) -> Sign/1, Abs1/1
  [Fn_strut] -> Calc Tire Force/3(Fn)
  [LocMatrix] -> Calc Tire Force/2(LocMatrix)
  [LocMatrix] -> Forces and distances to LMN/2(Xg_gnd)
  LocMatrix/1(A) -> [LocMatrix]
  [ZgB_prime] -> LocMatrix/2(ZgB_prime)
  [GearLoc] -> LocMatrix/1(XgB)
  Forces and distances to LMN/1(LMNe) -> Mux2/2
  Gear Local Force vector/1 -> Local Forces to Body Axes/2
  [Fn_strut] -> Gear Local Force vector/2
  Local Forces to Body Axes/1 -> Mux2/1, Forces and distances to LMN/1(Fb)
  [DCM] -> Local Forces to Body Axes/1
  [DCM] -> Calc Gear Force and Pos/4(DCM)
  [GearLoc] -> Calc Gear Force and Pos/3(Xg)
  Calc Gear Force and Pos/2(Fn_strut) -> [Fn_strut]
  [ZcL] -> Calc Gear Force and Pos/2(ZcL)
  Calc Gear Force and Pos/3(ZgB_prime) -> [ZgB_prime]
  Bus Selector3/1 -> Subsystem/1(Euler)  "<phi_theta_psi>"
  Subsystem/1(DCM) -> [DCM]

== system asbhl20vehicle/Vehicle/LandingGear GroundReaction/Nose Gear Geometry Forces and Moments/Subsystem ==
  Euler : Inport
  Bias : Bias  Bias=[0.0 0.0 -heading0*pi/180]
  Rotation Angles to Direction Cosine Matrix : aerolibtransform2/Rotation Angles to Direction Cosine Matrix  rotationOrder=ZYX
  Selector : Selector  InputPortWidth=3  IndexOptions=Index vector (dialog)  Indices=[3 2 1]  OutputSizes=1
  DCM : Outport
  wires:
  Bias/1 -> Selector/1
  Euler/1 -> Bias/1
  Rotation Angles to Direction Cosine Matrix/1 -> DCM/1
  Selector/1 -> Rotation Angles to Direction Cosine Matrix/1

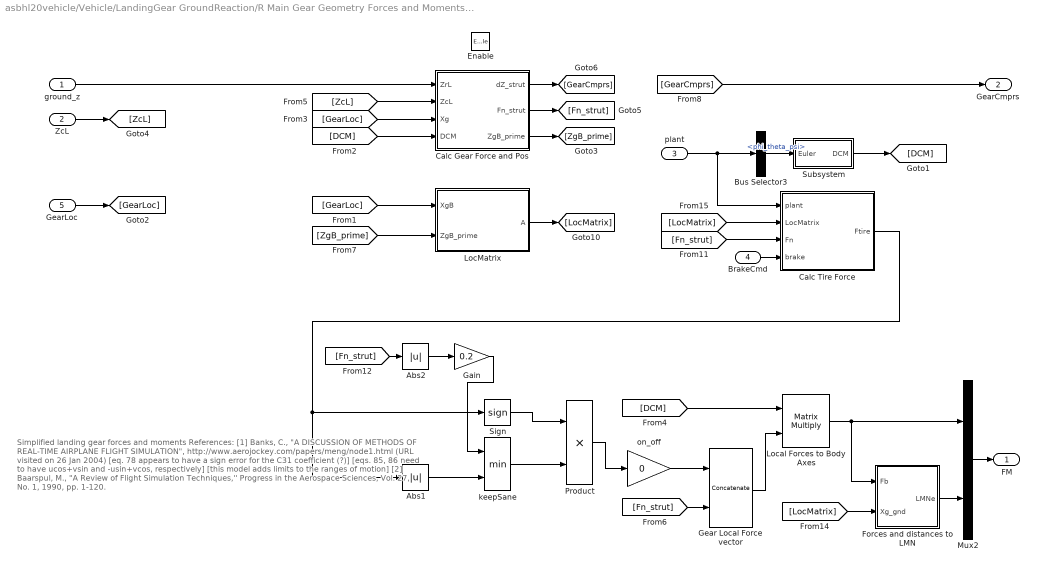
== system asbhl20vehicle/Vehicle/LandingGear GroundReaction/R Main Gear Geometry Forces and Moments/GenerateGroundFM ==
  note: Simplified landing gear forces and moments
      |
      | References:
      |
      | [1] Banks, C., "A DISCUSSION OF METHODS OF REAL-TIME AIRPLANE FLIGHT SIMULATION",
      | http://www.aerojockey.com/papers/meng/node1.html (URL visited on 26 Jan 2004)
      | [eq. 78 appears to have a sign error for the C31 coefficient (?)]
      | [eqs. 85, 86 need to have ucos+vsin and -usin+vcos, respectively]
      | [this model adds limits to the ranges of motion]
      |
      | [2] Baarspul, M., "A Review of Flight Simulation Techniques,''
      | Progress in the Aerospace Sciences, Vol. 27, No. 1, 1990, pp. 1-120.
  ground_z : Inport
  ZcL : Inport  Port=2
  plant : Inport  Port=3
  BrakeCmd : Inport  Port=4
  GearLoc : Inport  Port=5
  Enable : EnablePort  StatesWhenEnabling=reset
  Abs1 : Abs
  Abs2 : Abs
  Bus Selector3 : BusSelector  OutputSignals=phi_theta_psi
  Calc Gear Force and Pos : Subsystem
  Calc Tire Force : Subsystem
  Forces and distances to LMN : Subsystem
  Gain : Gain  Gain=0.2
  Gear Local Force vector : Concatenate  Mode=Multidimensional array
  LocMatrix : Subsystem
  Local Forces to Body Axes : Product  Multiplication=Matrix(*)  SaturateOnIntegerOverflow=on  InputSameDT=on  OutDataTypeStr=Inherit: Same as first input
  Mux2 : Mux  Inputs=2
  Product : Product  RndMeth=Zero
  Sign : Signum
  Subsystem : Subsystem
  keepSane : MinMax  Inputs=2
  on_off : Gain  Gain=0
  FM : Outport  PortDimensions=6  OutputWhenDisabled=reset  InitialOutput=[0,0,0,0,0,0]
  GearCmprs : Outport  Port=2  OutputWhenDisabled=reset  InitialOutput=0
  wires:
  Calc Gear Force and Pos/3(ZgB_prime) -> [ZgB_prime]
  [ZcL] -> Calc Gear Force and Pos/2(ZcL)
  Calc Gear Force and Pos/2(Fn_strut) -> [Fn_strut]
  [GearLoc] -> Calc Gear Force and Pos/3(Xg)
  [DCM] -> Calc Gear Force and Pos/4(DCM)
  [DCM] -> Local Forces to Body Axes/1
  Local Forces to Body Axes/1 -> Forces and distances to LMN/1(Fb), Mux2/1
  [Fn_strut] -> Gear Local Force vector/2
  Gear Local Force vector/1 -> Local Forces to Body Axes/2
  Forces and distances to LMN/1(LMNe) -> Mux2/2
  [GearLoc] -> LocMatrix/1(XgB)
  [ZgB_prime] -> LocMatrix/2(ZgB_prime)
  LocMatrix/1(A) -> [LocMatrix]
  [LocMatrix] -> Forces and distances to LMN/2(Xg_gnd)
  [LocMatrix] -> Calc Tire Force/2(LocMatrix)
  [Fn_strut] -> Calc Tire Force/3(Fn)
  Calc Tire Force/1(Ftire) -> Abs1/1, Sign/1
  on_off/1 -> Gear Local Force vector/1
  [Fn_strut] -> Abs2/1
  Abs2/1 -> Gain/1
  Gain/1 -> keepSane/1
  Abs1/1 -> keepSane/2
  keepSane/1 -> Product/2
  Product/1 -> on_off/1
  Sign/1 -> Product/1
  Calc Gear Force and Pos/1(dZ_strut) -> [GearCmprs]
  ground_z/1 -> Calc Gear Force and Pos/1(ZrL)
  plant/1 -> Bus Selector3/1, Calc Tire Force/1(plant)
  BrakeCmd/1 -> Calc Tire Force/4(brake)
  Mux2/1 -> FM/1
  GearLoc/1 -> [GearLoc]
  ZcL/1 -> [ZcL]
  [GearCmprs] -> GearCmprs/1
  Subsystem/1(DCM) -> [DCM]
  Bus Selector3/1 -> Subsystem/1(Euler)  "<phi_theta_psi>"

== system asbhl20vehicle/Vehicle/LandingGear GroundReaction/R Main Gear Geometry Forces and Moments/Subsystem1 ==
  Euler : Inport
  Bias : Bias  Bias=[0.0 0.0 -heading0*pi/180]
  Rotation Angles to Direction Cosine Matrix : aerolibtransform2/Rotation Angles to Direction Cosine Matrix  rotationOrder=ZYX
  Selector : Selector  InputPortWidth=3  IndexOptions=Index vector (dialog)  Indices=[3 2 1]  OutputSizes=1
  DCM : Outport
  wires:
  Bias/1 -> Selector/1
  Euler/1 -> Bias/1
  Rotation Angles to Direction Cosine Matrix/1 -> DCM/1
  Selector/1 -> Rotation Angles to Direction Cosine Matrix/1

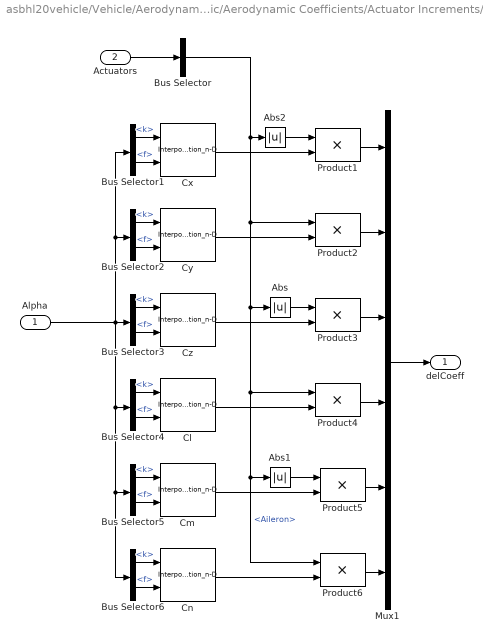
== system asbhl20vehicle/Vehicle/Aerodynamic/Aerodynamic Coefficients/Actuator Increments/Aileron ==
  Alpha : Inport
  Actuators : Inport  Port=2
  Abs : Abs  SaturateOnIntegerOverflow=on
  Abs1 : Abs  SaturateOnIntegerOverflow=on
  Abs2 : Abs  SaturateOnIntegerOverflow=on
  Bus Selector : BusSelector  OutputSignals=Aileron
  Bus Selector{1..6} (6 alike) : BusSelector  OutputSignals=k,f
  Cl : Interpolation_n-D  NumberOfTableDimensions=1  Table=Clda  RemoveProtectionIndex=on  SaturateOnIntegerOverflow=on
      settings: InputPortMap=u0,u1
  Cm : Interpolation_n-D  NumberOfTableDimensions=1  Table=Cmda  RemoveProtectionIndex=on  SaturateOnIntegerOverflow=on
      settings: InputPortMap=u0,u1
  Cn : Interpolation_n-D  NumberOfTableDimensions=1  Table=Cnda  RemoveProtectionIndex=on  SaturateOnIntegerOverflow=on
      settings: InputPortMap=u0,u1
  Cx : Interpolation_n-D  NumberOfTableDimensions=1  Table=CXda  RemoveProtectionIndex=on  SaturateOnIntegerOverflow=on
      settings: InputPortMap=u0,u1
  Cy : Interpolation_n-D  NumberOfTableDimensions=1  Table=CYda  RemoveProtectionIndex=on  SaturateOnIntegerOverflow=on
      settings: InputPortMap=u0,u1
  Cz : Interpolation_n-D  NumberOfTableDimensions=1  Table=CZda  RemoveProtectionIndex=on  SaturateOnIntegerOverflow=on
      settings: InputPortMap=u0,u1
  Mux1 : Mux  Inputs=6
  Product{1..6} (6 alike) : Product  SaturateOnIntegerOverflow=on  InputSameDT=on  OutDataTypeStr=Inherit: Same as first input
  delCoeff : Outport
  wires:
  Actuators/1 -> Bus Selector/1
  Mux1/1 -> delCoeff/1
  Product1/1 -> Mux1/1
  Cx/1 -> Product1/2
  Product2/1 -> Mux1/2
  Cy/1 -> Product2/2
  Product3/1 -> Mux1/3
  Cz/1 -> Product3/2
  Cl/1 -> Product4/2
  Product4/1 -> Mux1/4
  Cm/1 -> Product5/2
  Product5/1 -> Mux1/5
  Cn/1 -> Product6/2
  Product6/1 -> Mux1/6
  Bus Selector/1 -> Product6/1, Abs1/1, Product4/1, Abs/1, Product2/1, Abs2/1  "<Aileron>"
  Abs/1 -> Product3/1
  Abs1/1 -> Product5/1
  Abs2/1 -> Product1/1
  Alpha/1 -> Bus Selector1/1, Bus Selector2/1, Bus Selector5/1, Bus Selector6/1, Bus Selector4/1, Bus Selector3/1
  Bus Selector1/1 -> Cx/1  "<k>"
  Bus Selector1/2 -> Cx/2  "<f>"
  Bus Selector2/1 -> Cy/1  "<k>"
  Bus Selector2/2 -> Cy/2  "<f>"
  Bus Selector3/1 -> Cz/1  "<k>"
  Bus Selector3/2 -> Cz/2  "<f>"
  Bus Selector4/1 -> Cl/1  "<k>"
  Bus Selector4/2 -> Cl/2  "<f>"
  Bus Selector5/1 -> Cm/1  "<k>"
  Bus Selector5/2 -> Cm/2  "<f>"
  Bus Selector6/1 -> Cn/1  "<k>"
  Bus Selector6/2 -> Cn/2  "<f>"

== system asbhl20vehicle/Vehicle/Aerodynamic/Aerodynamic Coefficients/Actuator Increments/Elevator ==
  Alpha : Inport
  Actuators : Inport  Port=2
  Bus Selector1 : BusSelector  OutputSignals=Elevator
  Bus Selector2 : BusSelector  OutputSignals=k,f
  Bus Selector3 : BusSelector  OutputSignals=k,f
  Bus Selector5 : BusSelector  OutputSignals=k,f
  Cm : Interpolation_n-D  NumberOfTableDimensions=1  Table=Cmde  RemoveProtectionIndex=on  SaturateOnIntegerOverflow=on
      settings: InputPortMap=u0,u1
  Constant1 : Constant  Value=0
  Cx : Interpolation_n-D  NumberOfTableDimensions=1  Table=CXde  RemoveProtectionIndex=on  SaturateOnIntegerOverflow=on
      settings: InputPortMap=u0,u1
  Cz : Interpolation_n-D  NumberOfTableDimensions=1  Table=CZde  RemoveProtectionIndex=on  SaturateOnIntegerOverflow=on
      settings: InputPortMap=u0,u1
  Mux1 : Mux  Inputs=6
  Product : Product  SaturateOnIntegerOverflow=on  InputSameDT=on  OutDataTypeStr=Inherit: Same as first input
  delCoeff : Outport
  wires:
  Product/1 -> delCoeff/1
  Mux1/1 -> Product/1
  Alpha/1 -> Bus Selector2/1, Bus Selector3/1, Bus Selector5/1
  Cx/1 -> Mux1/1
  Cz/1 -> Mux1/3
  Cm/1 -> Mux1/5
  Constant1/1 -> Mux1/2, Mux1/4, Mux1/6
  Actuators/1 -> Bus Selector1/1
  Bus Selector1/1 -> Product/2  "<Elevator>"
  Bus Selector2/1 -> Cx/1  "<k>"
  Bus Selector2/2 -> Cx/2  "<f>"
  Bus Selector3/1 -> Cz/1  "<k>"
  Bus Selector3/2 -> Cz/2  "<f>"
  Bus Selector5/1 -> Cm/1  "<k>"
  Bus Selector5/2 -> Cm/2  "<f>"

== system asbhl20vehicle/Vehicle/Aerodynamic/Aerodynamic Coefficients/Actuator Increments/Flap(diff) ==
  Alpha : Inport
  Actuators : Inport  Port=2
  Abs2 : Abs  SaturateOnIntegerOverflow=on
  Bus Selector : BusSelector  OutputSignals=Flap(diff)
  Bus Selector{1..2,4,6} (4 alike) : BusSelector  OutputSignals=k,f
  Cl : Interpolation_n-D  NumberOfTableDimensions=1  Table=Clddf  RemoveProtectionIndex=on  SaturateOnIntegerOverflow=on
      settings: InputPortMap=u0,u1
  Cn : Interpolation_n-D  NumberOfTableDimensions=1  Table=Cnddf  RemoveProtectionIndex=on  SaturateOnIntegerOverflow=on
      settings: InputPortMap=u0,u1
  Constant1 : Constant  Value=0
  Cx : Interpolation_n-D  NumberOfTableDimensions=1  Table=CXddf  RemoveProtectionIndex=on  SaturateOnIntegerOverflow=on
      settings: InputPortMap=u0,u1
  Cy : Interpolation_n-D  NumberOfTableDimensions=1  Table=CYddf  RemoveProtectionIndex=on  SaturateOnIntegerOverflow=on
      settings: InputPortMap=u0,u1
  Mux1 : Mux  Inputs=6
  Product{,1..3} (4 alike) : Product  SaturateOnIntegerOverflow=on  InputSameDT=on  OutDataTypeStr=Inherit: Same as first input
  delCoeff : Outport
  wires:
  Mux1/1 -> delCoeff/1
  Alpha/1 -> Bus Selector4/1, Bus Selector6/1, Bus Selector1/1, Bus Selector2/1
  Actuators/1 -> Bus Selector/1
  Product/1 -> Mux1/1
  Cx/1 -> Product/2
  Bus Selector/1 -> Product3/1, Product2/1, Product1/1, Abs2/1  "<Flap(diff)>"
  Product1/1 -> Mux1/2
  Product2/1 -> Mux1/4
  Cl/1 -> Product2/2
  Cy/1 -> Product1/2
  Product3/1 -> Mux1/6
  Cn/1 -> Product3/2
  Abs2/1 -> Product/1
  Constant1/1 -> Mux1/3, Mux1/5
  Bus Selector1/1 -> Cx/1  "<k>"
  Bus Selector1/2 -> Cx/2  "<f>"
  Bus Selector2/1 -> Cy/1  "<k>"
  Bus Selector2/2 -> Cy/2  "<f>"
  Bus Selector4/1 -> Cl/1  "<k>"
  Bus Selector4/2 -> Cl/2  "<f>"
  Bus Selector6/1 -> Cn/1  "<k>"
  Bus Selector6/2 -> Cn/2  "<f>"

== system asbhl20vehicle/Vehicle/Aerodynamic/Aerodynamic Coefficients/Actuator Increments/Flap(neg) ==
  Alpha : Inport
  Actuators : Inport  Port=2
  Bus Selector : BusSelector  OutputSignals=Flap(neg)
  Bus Selector1 : BusSelector  OutputSignals=k,f
  Bus Selector3 : BusSelector  OutputSignals=k,f
  Bus Selector5 : BusSelector  OutputSignals=k,f
  Cm : Interpolation_n-D  NumberOfTableDimensions=1  Table=Cmdfn  RemoveProtectionIndex=on  SaturateOnIntegerOverflow=on
      settings: InputPortMap=u0,u1
  Constant1 : Constant  Value=0
  Constant2 : Constant  Value=0
  Constant3 : Constant  Value=0
  Cx : Interpolation_n-D  NumberOfTableDimensions=1  Table=CXdfn  RemoveProtectionIndex=on  SaturateOnIntegerOverflow=on
      settings: InputPortMap=u0,u1
  Cz : Interpolation_n-D  NumberOfTableDimensions=1  Table=CZdfn  RemoveProtectionIndex=on  SaturateOnIntegerOverflow=on
      settings: InputPortMap=u0,u1
  Mux1 : Mux  Inputs=6
  Product : Product  SaturateOnIntegerOverflow=on  InputSameDT=on  OutDataTypeStr=Inherit: Same as first input
  delCoeff : Outport
  wires:
  Cm/1 -> Mux1/5
  Cz/1 -> Mux1/3
  Cx/1 -> Mux1/1
  Alpha/1 -> Bus Selector5/1, Bus Selector3/1, Bus Selector1/1
  Mux1/1 -> Product/1
  Product/1 -> delCoeff/1
  Actuators/1 -> Bus Selector/1
  Constant1/1 -> Mux1/2
  Constant2/1 -> Mux1/4
  Constant3/1 -> Mux1/6
  Bus Selector/1 -> Product/2  "<Flap(neg)>"
  Bus Selector5/1 -> Cm/1  "<k>"
  Bus Selector5/2 -> Cm/2  "<f>"
  Bus Selector3/1 -> Cz/1  "<k>"
  Bus Selector3/2 -> Cz/2  "<f>"
  Bus Selector1/1 -> Cx/1  "<k>"
  Bus Selector1/2 -> Cx/2  "<f>"
